simulink model "huamo"  (R2014a)
settings: Solver=ode3  SolverMode=SingleTasking  StartTime=0.0  StopTime=10.0  RelTol=1e-3
PreLoadFcn:
  | waijung.modelPreload; % Required for working with Waijung Blockset. Do not remove.
undefined symbols (not defined in the file): ARM, dfilt, DiscIntNeverNeededParam, fdesignblkfcn, gcbh, Link, LQFP64, MDK, ST, STM32F405RG
libraries: simulink x33, stm32f4_io_lib x3, stm32f4_device_config_lib x2, dsparch4 x2
(part 6 of 6)

== system huamo/ from shangweiji/Enabled Subsystem1/If Action Subsystem1 ==
  Action Port : ActionPort  ActionType=else
  UART Tx : S-Function  Priority=1  FunctionName=stm32f4_usart  Parameters=configuration,uartmodule,transfer,baudrate,inputtype,outputtype,confstr,binheaderarray,binterminatorarray,asciiheader,asciiterminator,bindatalength,packetmode,varname,sampletime,sampletimestr,blockid  EnableBusSupport=off  mask(stm32f4_usart){configuration=Tx, uartmodule=1, baudrate=115200, databits=8, parity=No, stopbit=1, remaptxpin=Not used, remaprxpin=Not used, flowcontrol=None, remapctspin=Not used, remaprtspin=Not used, advanceoptions=off, rxbuffersize=512, txbuffersize=512, transfer=Non-Blocking, packetmode=Ascii, binheader='7E 7E', binterminator='03 03', porttype_double=0, porttype_single=0, porttype_int8=0, porttype_uint8=0, porttype_int16=0, porttype_uint16=0, porttype_int32=0, porttype_uint32=3, asciiformat='>>LED1 ON', rx_asciiterminator=CRLF (0x0D 0x0A - "\r\n"), tx_asciiterminator=CRLF (0x0D 0x0A - "\r\n"), storagename=<empty>, varname=, inputtype=[0 ], outputtype=[0], binheaderarray=[0], binterminatorarray=[0], bindatalength=0, asciiheader='>>LED1 ON\r\n', asciiterminator=[2 13 10], sampletime=1, sampletimestr=1, blockid=fromshangweijiEnabledSubsystem1IfActionSubsystem1UARTTx, confstr=[ "dummy", "0", "*", "*", "0", "*", "*", "0", "*", "*", "0", "*", "*", "2", "4", "7", "2", "4", "2", "512", "512", "2", "1", "115200", "8", "No", "1", "None", "USART1"], lastmodule=1}
      mask prompts: uartmodule "UART Module"; baudrate "Baud rate (bps)"; databits "Data bits"; stopbit "Stop bit"; remaptxpin "Tx Pin"; remaprxpin "Rx Pin"; flowcontrol "Hardware flow control"; remapctspin "HW Flow control, CTS Pin"; remaprtspin "HW Flow control, RTS Pin"; advanceoptions "Advance options"; rxbuffersize "Rx buffer size (bytes)"; txbuffersize "Tx buffer size (bytes)"; packetmode "Packet mode"; binheader "Binary header (example: '7E 7E')"; binterminator "Binary terminator (example: '03 03')"; porttype_double "Number of data port, type DOUBLE"; porttype_single "Number of data port, type SINGLE"; porttype_int8 "Number of data port, type INT8"; porttype_uint8 "Number of data port, type UINT8"; porttype_int16 "Number of data port, type INT16"; porttype_uint16 "Number of data port, type UINT16"; porttype_int32 "Number of data port, type INT32"; porttype_uint32 "Number of data port, type UINT32"; asciiformat "Ascii format"; rx_asciiterminator "End of packet"; tx_asciiterminator "End of packet"; storagename "Buffer"; varname "Var name"; inputtype "Input data type"; outputtype "Output data type"; binheaderarray "Binary header"; binterminatorarray "Binary terminator"; bindatalength "Binary data length"; asciiheader "Ascii header (printf format)"; asciiterminator "Ascii terminator"; sampletime "Sample time (sec)"; sampletimestr "Compiled sample time (sec) in string"; confstr "Configuration string"; lastmodule "Last module selected"
      mask help:
      | Data type for Ascii format
      | %u, %i, %d, %o, %x: uint32
      | %e, %g, %f: single
      | %c: int8
      mask init:
      | stm32f4_usart_callback('init');
      mask Help: web(fullfile(waijungdocroot,'stm32f4_usart_tx.htm'), '-browser')
      mask TypeOptions configuration: Setup | Tx | Rx
      mask Callback configuration: stm32f4_usart_callback('configuration');
      mask TypeOptions uartmodule: 1 | 2 | 3 | 4 | 5 | 6
      mask Callback uartmodule: stm32f4_usart_callback('uartmodule');
      mask Callback baudrate: stm32f4_usart_callback('baudrate');
      mask TypeOptions databits: 8
      mask TypeOptions parity: No | Odd | Even
      mask TypeOptions stopbit: 0.5 | 1 | 1.5 | 2
      mask TypeOptions remaptxpin: Not used | A9 | B6
      mask TypeOptions remaprxpin: Not used | A10 | B7
      mask TypeOptions flowcontrol: None | RTS | CTS | RTS/CTS
      mask Callback flowcontrol: stm32f4_usart_callback('flowcontrol');
      mask TypeOptions remapctspin: Not used | A11
      mask TypeOptions remaprtspin: Not used | A12
      mask Callback advanceoptions: stm32f4_usart_callback('advanceoptions');
      mask TypeOptions rxbuffersize: 16 | 32 | 64 | 128 | 256 | 512 | 1024 | 2048
      mask TypeOptions txbuffersize: 16 | 32 | 64 | 128 | 256 | 512 | 1024 | 2048
      mask TypeOptions transfer: Blocking | Non-Blocking
      mask Callback transfer: stm32f4_usart_callback('transfer');
      mask TypeOptions packetmode: Ascii | Binary | Binary Vector | String Buffer
      mask Callback packetmode: stm32f4_usart_callback('packetmode');
      mask Callback binheader: stm32f4_usart_callback('binheader');
      mask Callback binterminator: stm32f4_usart_callback('binterminator');
      mask Callback porttype_double: stm32f4_usart_callback('porttype');
      mask Callback porttype_single: stm32f4_usart_callback('porttype');
      mask Callback porttype_int8: stm32f4_usart_callback('porttype');
      mask Callback porttype_uint8: stm32f4_usart_callback('porttype');
      mask Callback porttype_int16: stm32f4_usart_callback('porttype');
      mask Callback porttype_uint16: stm32f4_usart_callback('porttype');
      mask Callback porttype_int32: stm32f4_usart_callback('porttype');
      mask Callback porttype_uint32: stm32f4_usart_callback('porttype');
      mask Callback asciiformat: stm32f4_usart_callback('asciiformat');
      mask TypeOptions rx_asciiterminator: CR (0x0D - "\r") | LF (0x0A - "\n") | CRLF (0x0D 0x0A - "\r\n")
      mask Callback rx_asciiterminator: stm32f4_usart_callback('rx_asciiterminator');
      mask TypeOptions tx_asciiterminator: CR (0x0D - "\r") | LF (0x0A - "\n") | CRLF (0x0D 0x0A - "\r\n") | None
      mask Callback tx_asciiterminator: stm32f4_usart_callback('tx_asciiterminator');
      mask TypeOptions storagename: <empty>
      mask Callback storagename: stm32f4_usart_callback('storagename');
      mask Callback varname: stm32f4_usart_callback('varname');
      mask Callback sampletime: stm32f4_usart_callback('sampletime');
      mask Callback sampletimestr: stm32f4_usart_callback('sampletimestr');
      mask Callback blockid: stm32f4_usart_callback('blockid');
      mask Display: text(0.5, 0.5, 'Module: USART1_Tx\nPacket: Ascii\nTransfer: Non-Blocking\nTs (sec): 1','ver','middle','hor','center');

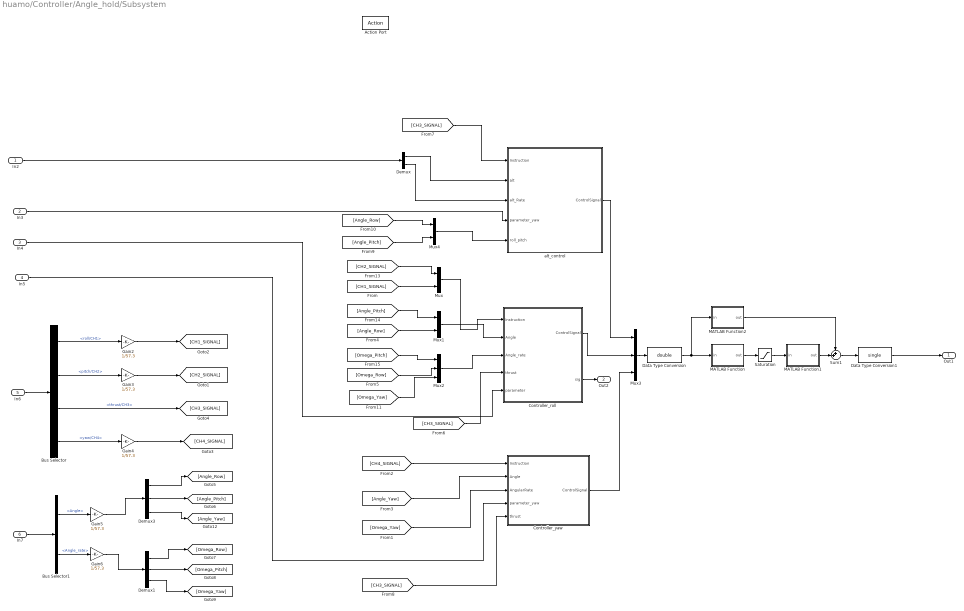
== system huamo/Controller/Angle_hold/Subsystem ==
  In2 : Inport
  In3 : Inport  Port=2
  In4 : Inport  Port=3
  In5 : Inport  Port=4
  In6 : Inport  Port=5
  In7 : Inport  Port=6
  Action Port : ActionPort  ActionType=then
  Bus Selector : BusSelector  OutputSignals=roll/CH1,pitch/CH2,thrust/CH3,yaw/CH4
  Bus Selector1 : BusSelector  OutputSignals=Angle,Angle_rate
  Controller_roll : Subsystem
  Controller_yaw : Subsystem
  Data Type Conversion : DataTypeConversion  OutDataTypeStr=double
  Data Type Conversion1 : DataTypeConversion  OutDataTypeStr=single
  Demux : Demux  Outputs=2
  Demux1 : Demux  Outputs=3
  Demux3 : Demux  Outputs=3
  Gain{2..6} (5 alike) : Gain  Gain=1/57.3
  MATLAB Function : MATLAB Function  TreatAsAtomicUnit=on
  MATLAB Function1 : MATLAB Function  TreatAsAtomicUnit=on
  MATLAB Function2 : MATLAB Function  TreatAsAtomicUnit=on
  Mux : Mux  Inputs=2
  Mux1 : Mux  Inputs=2
  Mux2 : Mux  Inputs=3
  Mux3 : Mux  Inputs=3
  Mux4 : Mux  Inputs=2
  Saturation : Saturate  UpperLimit=5.1564e+05  LowerLimit=8.0569e+03
  Sum1 : Sum  Inputs=++|
  alt_control : Subsystem
  Out1 : Outport
  Out2 : Outport  Port=2
  wires:
  In7/1 -> Bus Selector1/1
  Bus Selector1/2 -> Gain6/1  "<Angle_rate>"
  Bus Selector/4 -> Gain4/1  "<yaw/CH4>"
  In6/1 -> Bus Selector/1
  Bus Selector/2 -> Gain3/1  "<pitch/CH2>"
  Bus Selector/1 -> Gain2/1  "<roll/CH1>"
  Bus Selector/3 -> [CH3_SIGNAL]  "<thrust/CH3>"
  Demux3/1 -> [Angle_Row]
  Demux3/2 -> [Angle_Pitch]
  Demux1/1 -> [Omega_Row]
  Demux1/2 -> [Omega_Pitch]
  Demux1/3 -> [Omega_Yaw]
  Bus Selector1/1 -> Gain5/1  "<Angle>"
  Mux/1 -> Controller_roll/1(Instruction)
  Mux2/1 -> Controller_roll/3(Angle_rate)
  Mux1/1 -> Controller_roll/2(Angle)
  Demux3/3 -> [Angle_Yaw]
  [CH4_SIGNAL] -> Controller_yaw/1(Instruction)
  Gain2/1 -> [CH1_SIGNAL]
  Gain3/1 -> [CH2_SIGNAL]
  Gain4/1 -> [CH4_SIGNAL]
  Gain5/1 -> Demux3/1
  Gain6/1 -> Demux1/1
  Controller_yaw/1(ControlSignal) -> Mux3/3
  [Omega_Yaw] -> Controller_yaw/3(AngularRate)
  [Angle_Yaw] -> Controller_yaw/2(Angle)
  Mux3/1 -> Data Type Conversion/1
  MATLAB Function/1(out) -> Saturation/1
  Data Type Conversion/1 -> MATLAB Function2/1(in), MATLAB Function/1(in)
  Data Type Conversion1/1 -> Out1/1
  Saturation/1 -> MATLAB Function1/1(in)
  In4/1 -> Controller_roll/5(parameter)
  In5/1 -> Controller_yaw/4(parameter_yaw)
  [CH3_SIGNAL] -> Controller_roll/4(thrust)
  [CH3_SIGNAL] -> Controller_yaw/5(thrust)
  In2/1 -> Demux/1
  Demux/1 -> alt_control/2(alt)
  Demux/2 -> alt_control/3(alt_Rate)
  In3/1 -> alt_control/4(parameter_yaw)
  [Angle_Row] -> Mux4/1
  [Angle_Pitch] -> Mux4/2
  Mux4/1 -> alt_control/5(roll_pitch)
  alt_control/1(ControlSignal) -> Mux3/1
  [Omega_Row] -> Mux2/2
  [Omega_Pitch] -> Mux2/1
  [Angle_Row] -> Mux1/2
  [Angle_Pitch] -> Mux1/1
  [CH1_SIGNAL] -> Mux/2
  [CH2_SIGNAL] -> Mux/1
  Controller_roll/1(ControlSignal) -> Mux3/2
  Sum1/1 -> Data Type Conversion1/1
  MATLAB Function1/1(out) -> Sum1/2
  MATLAB Function2/1(out) -> Sum1/1
  Controller_roll/2(sig) -> Out2/1
  [CH3_SIGNAL] -> alt_control/1(Instruction)
  [Omega_Yaw] -> Mux2/3

== system huamo/Controller/Velocity_Damper1/Altitude_calculation ==
  Accelerometer : Inport
  Barometer : Inport  Port=2
  Basic_altitude : Inport  Port=3
  Enable : EnablePort
  Data Type Conversion : DataTypeConversion  OutDataTypeStr=single
  Data Type Conversion1 : DataTypeConversion  OutDataTypeStr=single
  Demux : Demux  Outputs=3
  Digital Clock : DigitalClock  SampleTime=-1
  Discrete-Time Integrator : DiscreteIntegrator  gainval=1  SampleTime=-1  ICPrevOutput=DiscIntNeverNeededParam  ICPrevScaledInput=DiscIntNeverNeededParam
  Discrete-Time Integrator1 : DiscreteIntegrator  SampleTime=-1  ICPrevOutput=DiscIntNeverNeededParam  ICPrevScaledInput=DiscIntNeverNeededParam
  Divide : Product  Inputs=**
  Gain2 : Gain  Gain=0.45
  Gain3 : Gain  Gain=0.65
  MATLAB Function : MATLAB Function  TreatAsAtomicUnit=on
  Rate Transition : RateTransition
  Sum{1..4} (4 alike) : Sum  Inputs=|+-
  Terminator : Terminator
  Terminator1 : Terminator
  Out1 : Outport
  wires:
  Rate Transition/1 -> Sum1/2
  Discrete-Time Integrator1/1 -> Out1/1, Sum1/1
  Discrete-Time Integrator/1 -> Sum3/1
  Sum4/1 -> Discrete-Time Integrator/1
  Sum3/1 -> Discrete-Time Integrator1/1
  Sum2/1 -> Rate Transition/1
  Demux/3 -> Sum4/1
  Barometer/1 -> Sum2/1
  Basic_altitude/1 -> Data Type Conversion/1
  Data Type Conversion/1 -> Sum2/2
  Accelerometer/1 -> Demux/1
  Demux/1 -> Terminator/1
  Demux/2 -> Terminator1/1
  Gain2/1 -> Sum4/2
  Gain3/1 -> Sum3/2
  Divide/1 -> Gain2/1, Gain3/1
  Sum1/1 -> Divide/1
  MATLAB Function/1(y) -> Data Type Conversion1/1
  Digital Clock/1 -> MATLAB Function/1(u)
  Data Type Conversion1/1 -> Divide/2

== system huamo/Controller/Velocity_Damper1/Controller ==
  In1 : Inport
  Discrete Derivative : simulink/Discrete/Discrete Derivative  gainval=1.0  ICPrevScaledInput=0.0  InputProcessing=Inherited  OutMin=[]  OutMax=[]  OutDataType=fixdt(1, 16)  OutScaling=2^-10  DoSatur=off
  Discrete FIR Filter : DiscreteFir  SampleTime=0.05
  Saturation : Saturate  UpperLimit=2  LowerLimit=-2
  Out1 : Outport
  wires:
  In1/1 -> Discrete Derivative/1
  Discrete Derivative/1 -> Discrete FIR Filter/1
  Saturation/1 -> Out1/1
  Discrete FIR Filter/1 -> Saturation/1

== system huamo/Controller/Velocity_Damper1/Horizontal_velocity ==
  note: To get true velocity ,the output of the loop needs to multiply -1
  In1 : Inport
  Dead Zone : DeadZone  LowerValue=-0.15  UpperValue=0.15  SaturateOnIntegerOverflow=on
  Demux : Demux  Outputs=3
  Discrete-Time Integrator : DiscreteIntegrator  SampleTime=-1  ICPrevOutput=DiscIntNeverNeededParam  ICPrevScaledInput=DiscIntNeverNeededParam
  Gain : Gain  Gain=0.5
  Gain2 : Gain  Gain=20
  Gain4 : Gain  Gain=-1
  Saturation : Saturate  UpperLimit=20  LowerLimit=-20
  Sum : Sum  Inputs=|+-
  Terminator : Terminator
  Out1 : Outport
  Out2 : Outport  Port=2
  wires:
  Demux/3 -> Terminator/1
  Demux/1 -> Out1/1
  Sum/1 -> Discrete-Time Integrator/1
  Gain/1 -> Sum/2
  Demux/2 -> Out2/1
  Discrete-Time Integrator/1 -> Gain4/1, Gain/1
  In1/1 -> Sum/1
  Dead Zone/1 -> Gain2/1
  Gain2/1 -> Saturation/1
  Saturation/1 -> Demux/1
  Gain4/1 -> Dead Zone/1

== system huamo/Controller/Velocity_Damper1/If Action Subsystem ==
  Action Port : ActionPort  ActionType=then
  Constant : Constant
  Out1 : Outport  InitialOutput=0
  wires:
  Constant/1 -> Out1/1

== system huamo/Controller/Velocity_Damper1/accb_to_acce ==
  angle : Inport
  accel : Inport  Port=2
  bias_acc : Inport  Port=3
  body axis to earth axis : MATLAB Function  TreatAsAtomicUnit=on
  Out1 : Outport
  wires:
  angle/1 -> body axis to earth axis/1(angle)
  accel/1 -> body axis to earth axis/2(acc_body)
  bias_acc/1 -> body axis to earth axis/3(bia_acc)
  body axis to earth axis/1(acc_earth) -> Out1/1

== system huamo/Controller/Velocity_Damper2/Controller ==
  In1 : Inport
  Discrete Derivative : simulink/Discrete/Discrete Derivative  gainval=1.0  ICPrevScaledInput=0.0  InputProcessing=Inherited  OutMin=[]  OutMax=[]  OutDataType=fixdt(1, 16)  OutScaling=2^-10  DoSatur=off
  Lowpass Filter : Subsystem  DialogController=fdesignblkfcn  InitFcn=fdesignblkfcn(gcbh, {'InitFcn'});  mask(Lowpass Filter){}
      mask help: Design a lowpass filter
      settings: CopyFcn=fdesignblkfcn(gcbh, {'CopyFcn'});
      mask Help: helpview(mapfilelocation('dsp'), 'dsplowpassfilter');
      mask Display: disp('Lowpass')
  Saturation : Saturate  UpperLimit=2  LowerLimit=-2
  Out1 : Outport
  wires:
  In1/1 -> Discrete Derivative/1
  Discrete Derivative/1 -> Lowpass Filter/1(In)
  Saturation/1 -> Out1/1
  Lowpass Filter/1(Out) -> Saturation/1

== system huamo/Controller/Velocity_Damper2/Lowpass Filter ==
  In : Inport
  Generated Filter Block : dsparch4/Biquad Filter  Tag=BlockMethodSubSystem  IIRFiltStruct=Direct form II  CoeffSource=Specify via dialog  BiQuadCoeffs=[0.31598662750883372 0.36803820725630498 0.31598662750883377 1 -1.8265775363780477 0.840471451002894]  a0Flag=Warning  IC=0  ICnum=0  ICden=0  InputProcessing=Columns as channels (frame based)  denAccumFracLength=30  denProdOutputFracLength=30  secondMemoryFracLength=15  roundingMode=Floor  overflowMode=off  ScaleValues=[0.013893755370815749;1]  optimizeScaleValues=off  ScaleValueMode=Specify via input port (g)  scaleValueFracLength=14  FilterSource=Specify via dialog  dfiltObjectName=dfilt.df2tsos([1 0.3 0.4],[1 0.1 0.2])
  Out : Outport
  wires:
  In/1 -> Generated Filter Block/1
  Generated Filter Block/1 -> Out/1

== system huamo/IMU/Cal/bu ma ==
  In1 : Inport
  Bitwise Operator : simulink/Logic and Bit Operations/Bitwise Operator  logicop=NOT  UseBitMask=off  BitMask=bin2dec('11011001')  BitMaskRealWorld=Stored Integer
  Bitwise Operator1 : simulink/Logic and Bit Operations/Bitwise Operator  logicop=OR  UseBitMask=on  BitMask=bin2dec('1000000000000000')  BitMaskRealWorld=Stored Integer
  Bitwise Operator2 : simulink/Logic and Bit Operations/Bitwise Operator  logicop=AND  UseBitMask=on  BitMask=bin2dec('1000000000000000')  BitMaskRealWorld=Stored Integer
  Constant : Constant  OutDataTypeStr=int16
  Sum : Sum  Inputs=|++
  Switch : Switch  Criteria=u2 > Threshold
  Out1 : Outport
  wires:
  Switch/1 -> Out1/1
  Bitwise Operator/1 -> Bitwise Operator1/1
  Constant/1 -> Sum/2
  Bitwise Operator1/1 -> Sum/1
  Sum/1 -> Switch/1
  In1/1 -> Bitwise Operator/1, Switch/3, Bitwise Operator2/1
  Bitwise Operator2/1 -> Switch/2

== system huamo/IMU/Cal/bu ma1 ==
  In1 : Inport
  Bitwise Operator : simulink/Logic and Bit Operations/Bitwise Operator  logicop=NOT  UseBitMask=off  BitMask=bin2dec('11011001')  BitMaskRealWorld=Stored Integer
  Bitwise Operator1 : simulink/Logic and Bit Operations/Bitwise Operator  logicop=OR  UseBitMask=on  BitMask=bin2dec('1000000000000000')  BitMaskRealWorld=Stored Integer
  Bitwise Operator2 : simulink/Logic and Bit Operations/Bitwise Operator  logicop=AND  UseBitMask=on  BitMask=bin2dec('1000000000000000')  BitMaskRealWorld=Stored Integer
  Constant : Constant  OutDataTypeStr=int16
  Sum : Sum  Inputs=|++
  Switch : Switch  Criteria=u2 > Threshold
  Out1 : Outport
  wires:
  Switch/1 -> Out1/1
  Bitwise Operator/1 -> Bitwise Operator1/1
  Constant/1 -> Sum/2
  Bitwise Operator1/1 -> Sum/1
  Sum/1 -> Switch/1
  In1/1 -> Bitwise Operator/1, Switch/3, Bitwise Operator2/1
  Bitwise Operator2/1 -> Switch/2

== system huamo/IMU/Cal/bu ma2 ==
  In1 : Inport
  Bitwise Operator : simulink/Logic and Bit Operations/Bitwise Operator  logicop=NOT  UseBitMask=off  BitMask=bin2dec('11011001')  BitMaskRealWorld=Stored Integer
  Bitwise Operator1 : simulink/Logic and Bit Operations/Bitwise Operator  logicop=OR  UseBitMask=on  BitMask=bin2dec('1000000000000000')  BitMaskRealWorld=Stored Integer
  Bitwise Operator2 : simulink/Logic and Bit Operations/Bitwise Operator  logicop=AND  UseBitMask=on  BitMask=bin2dec('1000000000000000')  BitMaskRealWorld=Stored Integer
  Constant : Constant  OutDataTypeStr=int16
  Sum : Sum  Inputs=|++
  Switch : Switch  Criteria=u2 > Threshold
  Out1 : Outport
  wires:
  Switch/1 -> Out1/1
  Bitwise Operator/1 -> Bitwise Operator1/1
  Constant/1 -> Sum/2
  Bitwise Operator1/1 -> Sum/1
  Sum/1 -> Switch/1
  In1/1 -> Bitwise Operator/1, Switch/3, Bitwise Operator2/1
  Bitwise Operator2/1 -> Switch/2

== system huamo/IMU/Cal/bu ma3 ==
  In1 : Inport
  Bitwise Operator : simulink/Logic and Bit Operations/Bitwise Operator  logicop=NOT  UseBitMask=off  BitMask=bin2dec('11011001')  BitMaskRealWorld=Stored Integer
  Bitwise Operator1 : simulink/Logic and Bit Operations/Bitwise Operator  logicop=OR  UseBitMask=on  BitMask=bin2dec('1000000000000000')  BitMaskRealWorld=Stored Integer
  Bitwise Operator2 : simulink/Logic and Bit Operations/Bitwise Operator  logicop=AND  UseBitMask=on  BitMask=bin2dec('1000000000000000')  BitMaskRealWorld=Stored Integer
  Constant : Constant  OutDataTypeStr=int16
  Sum : Sum  Inputs=|++
  Switch : Switch  Criteria=u2 > Threshold
  Out1 : Outport
  wires:
  Switch/1 -> Out1/1
  Bitwise Operator/1 -> Bitwise Operator1/1
  Constant/1 -> Sum/2
  Bitwise Operator1/1 -> Sum/1
  Sum/1 -> Switch/1
  In1/1 -> Bitwise Operator/1, Switch/3, Bitwise Operator2/1
  Bitwise Operator2/1 -> Switch/2

== system huamo/IMU/Cal/bu ma4 ==
  In1 : Inport
  Bitwise Operator : simulink/Logic and Bit Operations/Bitwise Operator  logicop=NOT  UseBitMask=off  BitMask=bin2dec('11011001')  BitMaskRealWorld=Stored Integer
  Bitwise Operator1 : simulink/Logic and Bit Operations/Bitwise Operator  logicop=OR  UseBitMask=on  BitMask=bin2dec('1000000000000000')  BitMaskRealWorld=Stored Integer
  Bitwise Operator2 : simulink/Logic and Bit Operations/Bitwise Operator  logicop=AND  UseBitMask=on  BitMask=bin2dec('1000000000000000')  BitMaskRealWorld=Stored Integer
  Constant : Constant  OutDataTypeStr=int16
  Sum : Sum  Inputs=|++
  Switch : Switch  Criteria=u2 > Threshold
  Out1 : Outport
  wires:
  Switch/1 -> Out1/1
  Bitwise Operator/1 -> Bitwise Operator1/1
  Constant/1 -> Sum/2
  Bitwise Operator1/1 -> Sum/1
  Sum/1 -> Switch/1
  In1/1 -> Bitwise Operator/1, Switch/3, Bitwise Operator2/1
  Bitwise Operator2/1 -> Switch/2

== system huamo/IMU/Cal/bu ma5 ==
  In1 : Inport
  Bitwise Operator : simulink/Logic and Bit Operations/Bitwise Operator  logicop=NOT  UseBitMask=off  BitMask=bin2dec('11011001')  BitMaskRealWorld=Stored Integer
  Bitwise Operator1 : simulink/Logic and Bit Operations/Bitwise Operator  logicop=OR  UseBitMask=on  BitMask=bin2dec('1000000000000000')  BitMaskRealWorld=Stored Integer
  Bitwise Operator2 : simulink/Logic and Bit Operations/Bitwise Operator  logicop=AND  UseBitMask=on  BitMask=bin2dec('1000000000000000')  BitMaskRealWorld=Stored Integer
  Constant : Constant  OutDataTypeStr=int16
  Sum : Sum  Inputs=|++
  Switch : Switch  Criteria=u2 > Threshold
  Out1 : Outport
  wires:
  Switch/1 -> Out1/1
  Bitwise Operator/1 -> Bitwise Operator1/1
  Constant/1 -> Sum/2
  Bitwise Operator1/1 -> Sum/1
  Sum/1 -> Switch/1
  In1/1 -> Bitwise Operator/1, Switch/3, Bitwise Operator2/1
  Bitwise Operator2/1 -> Switch/2

== system huamo/IMU/Cal/bu ma6 ==
  In1 : Inport
  Bitwise Operator : simulink/Logic and Bit Operations/Bitwise Operator  logicop=NOT  UseBitMask=off  BitMask=bin2dec('11011001')  BitMaskRealWorld=Stored Integer
  Bitwise Operator1 : simulink/Logic and Bit Operations/Bitwise Operator  logicop=OR  UseBitMask=on  BitMask=bin2dec('1000000000000000')  BitMaskRealWorld=Stored Integer
  Bitwise Operator2 : simulink/Logic and Bit Operations/Bitwise Operator  logicop=AND  UseBitMask=on  BitMask=bin2dec('1000000000000000')  BitMaskRealWorld=Stored Integer
  Constant : Constant  OutDataTypeStr=int16
  Sum : Sum  Inputs=|++
  Switch : Switch  Criteria=u2 > Threshold
  Out1 : Outport
  wires:
  Switch/1 -> Out1/1
  Bitwise Operator/1 -> Bitwise Operator1/1
  Constant/1 -> Sum/2
  Bitwise Operator1/1 -> Sum/1
  Sum/1 -> Switch/1
  In1/1 -> Bitwise Operator/1, Switch/3, Bitwise Operator2/1
  Bitwise Operator2/1 -> Switch/2

== system huamo/Controller/Angle_hold/Subsystem/Controller_roll ==
  Instruction : Inport
  Angle : Inport  Port=2
  Angle_rate : Inport  Port=3
  thrust : Inport  Port=4
  parameter : Inport  Port=5
  Data Type Conversion : DataTypeConversion  OutDataTypeStr=single
  Data Type Conversion8 : DataTypeConversion  OutDataTypeStr=double
  Mux1 : Mux  Inputs=5
  Saturation : Saturate  UpperLimit=0.8  LowerLimit=-0.8
  attitude_control : MATLAB Function  TreatAsAtomicUnit=on
  ControlSignal : Outport
  sig : Outport  Port=2
  wires:
  Data Type Conversion/1 -> Saturation/1
  Saturation/1 -> ControlSignal/1
  attitude_control/1(out) -> sig/1, Data Type Conversion/1
  Data Type Conversion8/1 -> attitude_control/1(in)
  Instruction/1 -> Mux1/1
  Angle/1 -> Mux1/2
  Angle_rate/1 -> Mux1/3
  thrust/1 -> Mux1/4
  parameter/1 -> Mux1/5
  Mux1/1 -> Data Type Conversion8/1

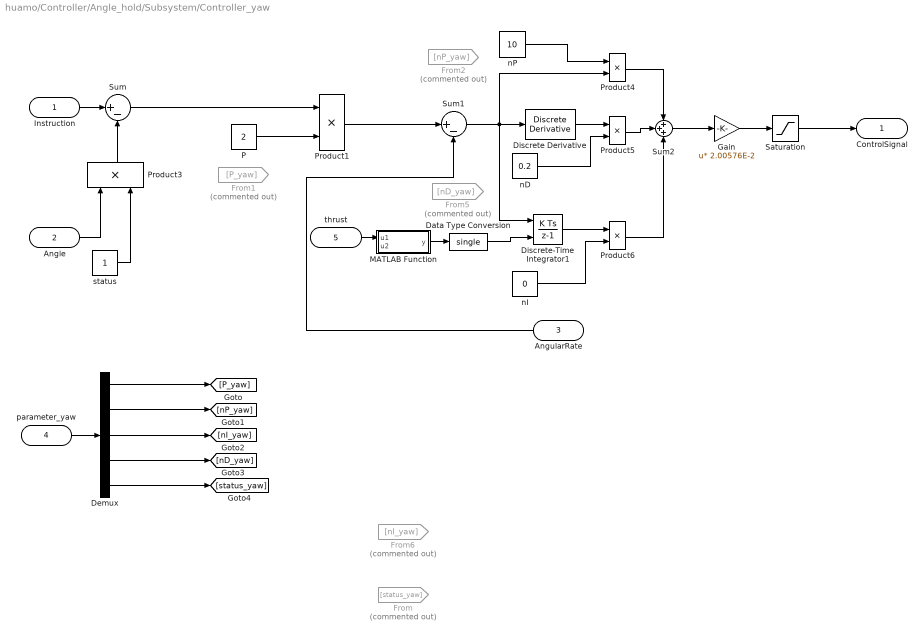
== system huamo/Controller/Angle_hold/Subsystem/Controller_yaw ==
  Instruction : Inport
  Angle : Inport  Port=2
  AngularRate : Inport  Port=3
  parameter_yaw : Inport  Port=4
  thrust : Inport  Port=5
  Data Type Conversion : DataTypeConversion  OutDataTypeStr=single
  Demux : Demux  Outputs=5
  Discrete Derivative : simulink/Discrete/Discrete Derivative  gainval=1.0  ICPrevScaledInput=0.01  InputProcessing=Inherited  OutMin=[]  OutMax=[]  OutDataType=fixdt(1, 16)  OutScaling=2^-10  DoSatur=off
  Discrete-Time Integrator1 : DiscreteIntegrator  ExternalReset=level  SampleTime=-1  LimitOutput=on  UpperSaturationLimit=2  LowerSaturationLimit=-2  ICPrevOutput=DiscIntNeverNeededParam  ICPrevScaledInput=DiscIntNeverNeededParam
  From : From  Commented=on  GotoTag=status_yaw
  From1 : From  Commented=on  GotoTag=P_yaw
  From2 : From  Commented=on  GotoTag=nP_yaw
  From5 : From  Commented=on  GotoTag=nD_yaw
  From6 : From  Commented=on  GotoTag=nI_yaw
  Gain : Gain  Gain=2.00576E-2  Multiplication=Matrix(u*K)  OutDataTypeStr=single
  MATLAB Function : MATLAB Function  TreatAsAtomicUnit=on
  P : Constant  Value=2  OutDataTypeStr=single
  Product{1,3..6} (5 alike) : Product
  Saturation : Saturate  UpperLimit=0.2  LowerLimit=-0.2
  Sum : Sum  Inputs=|+-
  Sum1 : Sum  Inputs=|+-  OutDataTypeStr=double
  Sum2 : Sum  Inputs=+++
  nD : Constant  Value=0.2  OutDataTypeStr=single
  nI : Constant  Value=0  OutDataTypeStr=single
  nP : Constant  Value=10  OutDataTypeStr=single
  status : Constant  OutDataTypeStr=single
  ControlSignal : Outport
  wires:
  Instruction/1 -> Sum/1
  Sum/1 -> Product1/1
  Sum1/1 -> Discrete Derivative/1, Discrete-Time Integrator1/1, Product4/2
  Angle/1 -> Product3/1
  Product3/1 -> Sum/2
  Sum2/1 -> Gain/1
  Discrete Derivative/1 -> Product5/1
  Discrete-Time Integrator1/1 -> Product6/1
  Product5/1 -> Sum2/2
  Product4/1 -> Sum2/1
  Product6/1 -> Sum2/3
  Product1/1 -> Sum1/1
  AngularRate/1 -> Sum1/2
  Gain/1 -> Saturation/1
  Saturation/1 -> ControlSignal/1
  parameter_yaw/1 -> Demux/1
  Demux/1 -> [P_yaw]
  Demux/2 -> [nP_yaw]
  Demux/3 -> [nI_yaw]
  Demux/4 -> [nD_yaw]
  Demux/5 -> [status_yaw]
  thrust/1 -> MATLAB Function/1(u1)
  MATLAB Function/1(y) -> Data Type Conversion/1
  Data Type Conversion/1 -> Discrete-Time Integrator1/2
  status/1 -> Product3/2
  nI/1 -> Product6/2
  nP/1 -> Product4/1
  P/1 -> Product1/2
  nD/1 -> Product5/2

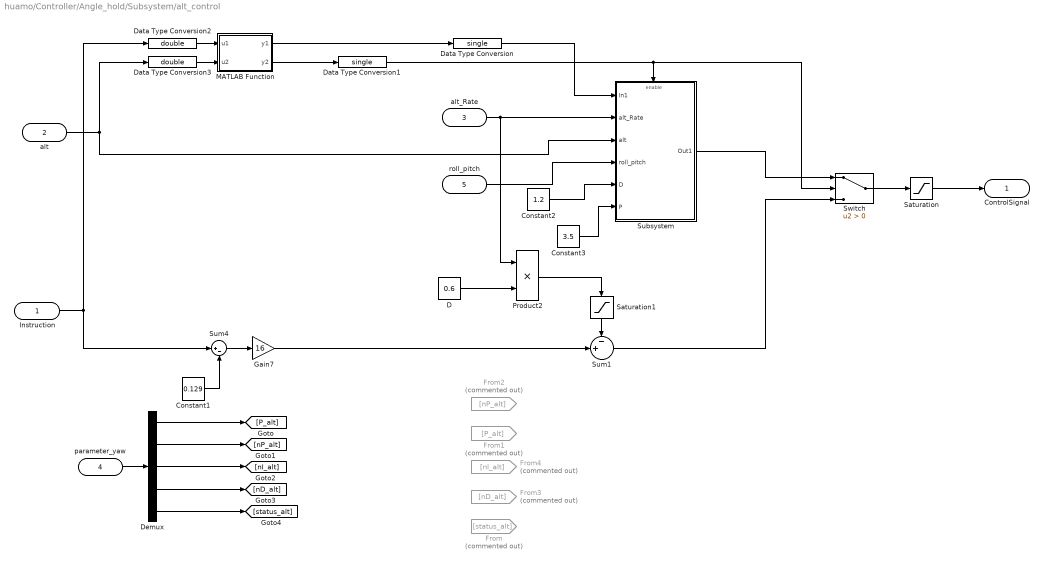
== system huamo/Controller/Angle_hold/Subsystem/alt_control ==
  Instruction : Inport
  alt : Inport  Port=2
  alt_Rate : Inport  Port=3
  parameter_yaw : Inport  Port=4
  roll_pitch : Inport  Port=5
  Constant1 : Constant  Value=0.129  OutDataTypeStr=single
  Constant2 : Constant  Value=1.2  OutDataTypeStr=single
  Constant3 : Constant  Value=3.5  OutDataTypeStr=single
  D : Constant  Value=0.6  OutDataTypeStr=single
  Data Type Conversion : DataTypeConversion  OutDataTypeStr=single
  Data Type Conversion1 : DataTypeConversion  OutDataTypeStr=single
  Data Type Conversion2 : DataTypeConversion  OutDataTypeStr=double
  Data Type Conversion3 : DataTypeConversion  OutDataTypeStr=double
  Demux : Demux  Outputs=5
  From : From  Commented=on  GotoTag=status_alt
  From1 : From  Commented=on  GotoTag=P_alt
  From2 : From  Commented=on  GotoTag=nP_alt
  From3 : From  Commented=on  GotoTag=nD_alt
  From4 : From  Commented=on  GotoTag=nI_alt
  Gain7 : Gain  Gain=16
  MATLAB Function : MATLAB Function  TreatAsAtomicUnit=on
  Product2 : Product
  Saturation : Saturate  UpperLimit=10  LowerLimit=0.272
  Saturation1 : Saturate  UpperLimit=1  LowerLimit=-1
  Subsystem : Subsystem
  Sum1 : Sum  Inputs=-+|  OutDataTypeStr=single
  Sum4 : Sum  Inputs=|+-
  Switch : Switch  Criteria=u2 > Threshold
  ControlSignal : Outport
  wires:
  Instruction/1 -> Sum4/1, Data Type Conversion2/1
  alt/1 -> Subsystem/3(alt), Data Type Conversion3/1
  Saturation/1 -> ControlSignal/1
  parameter_yaw/1 -> Demux/1
  Demux/1 -> [P_alt]
  Demux/2 -> [nP_alt]
  Demux/3 -> [nI_alt]
  Demux/4 -> [nD_alt]
  Demux/5 -> [status_alt]
  Constant1/1 -> Sum4/2
  Sum4/1 -> Gain7/1
  alt_Rate/1 -> Subsystem/2(alt_Rate), Product2/1
  roll_pitch/1 -> Subsystem/4(roll_pitch)
  MATLAB Function/1(y1) -> Data Type Conversion/1
  MATLAB Function/2(y2) -> Data Type Conversion1/1
  D/1 -> Product2/2
  Gain7/1 -> Sum1/2
  Product2/1 -> Saturation1/1
  Sum1/1 -> Switch/3
  Subsystem/1(Out1) -> Switch/1
  Switch/1 -> Saturation/1
  Data Type Conversion/1 -> Subsystem/1(In1)
  Data Type Conversion1/1 -> Subsystem/Enable, Switch/2
  Data Type Conversion2/1 -> MATLAB Function/1(u1)
  Data Type Conversion3/1 -> MATLAB Function/2(u2)
  Saturation1/1 -> Sum1/1
  Constant2/1 -> Subsystem/5(D)
  Constant3/1 -> Subsystem/6(P)

== system huamo/Controller/Velocity_Damper2/Controller/Lowpass Filter ==
  In : Inport
  Generated Filter Block : dsparch4/Biquad Filter  Tag=BlockMethodSubSystem  IIRFiltStruct=Direct form II  CoeffSource=Specify via dialog  BiQuadCoeffs=[0.31598662750883372 0.36803820725630498 0.31598662750883377 1 -1.8265775363780477 0.840471451002894]  a0Flag=Warning  IC=0  ICnum=0  ICden=0  InputProcessing=Columns as channels (frame based)  denAccumFracLength=30  denProdOutputFracLength=30  secondMemoryFracLength=15  roundingMode=Floor  overflowMode=off  ScaleValues=[0.013893755370815749;1]  optimizeScaleValues=off  ScaleValueMode=Specify via input port (g)  scaleValueFracLength=14  FilterSource=Specify via dialog  dfiltObjectName=dfilt.df2tsos([1 0.3 0.4],[1 0.1 0.2])
  Out : Outport
  wires:
  In/1 -> Generated Filter Block/1
  Generated Filter Block/1 -> Out/1

== system huamo/Controller/Angle_hold/Subsystem/alt_control/Subsystem ==
  In1 : Inport
  alt_Rate : Inport  Port=2
  alt : Inport  Port=3
  roll_pitch : Inport  Port=4
  D : Inport  Port=5
  P : Inport  Port=6
  Enable : EnablePort
  Constant : Constant  Value=10  OutDataTypeStr=single
  Constant1 : Constant  Value=0.43  OutDataTypeStr=single
  Data Type Conversion1 : DataTypeConversion  OutDataTypeStr=single
  Divide : Product  Inputs=*/  OutDataTypeStr=single
  Fcn : Fcn  Expr=cos(u(1))*cos(u(2))
  Product1 : Product
  Product2 : Product
  Product4 : Product
  Saturation1 : Saturate  UpperLimit=1.5  LowerLimit=-1.5
  Sum : Sum  Inputs=|+-
  Sum1 : Sum  Inputs=|+-  OutDataTypeStr=double
  Sum2 : Sum  Inputs=|++
  Out1 : Outport
  wires:
  alt_Rate/1 -> Product2/1
  Sum/1 -> Product1/1
  alt/1 -> Sum/2
  Product1/1 -> Sum1/1
  roll_pitch/1 -> Fcn/1
  Fcn/1 -> Data Type Conversion1/1
  Divide/1 -> Out1/1
  In1/1 -> Sum/1
  Data Type Conversion1/1 -> Divide/2
  Constant/1 -> Sum2/2
  Sum1/1 -> Sum2/1
  Constant1/1 -> Product4/2
  Sum2/1 -> Product4/1
  Product4/1 -> Divide/1
  Product2/1 -> Saturation1/1
  Saturation1/1 -> Sum1/2
  P/1 -> Product1/2
  D/1 -> Product2/2

== matlab function huamo/Receiver/Enabled Subsystem/MATLAB Function2 ==
  data: u input; y output
function y = fcn(u)
%#codegen
%输入范围为0.34~1.7，将其调整到1~2ms
    u=u/1.375+0.76;
    if (u>0.8)&&(u<2.1)
        y=u;
    else
        y=1.5;    
    end

== matlab function huamo/Receiver/Enabled Subsystem/MATLAB Function4 ==
  data: u input; y output
function y = fcn(u)
%#codegen
%输入范围为0.34~1.7，将其调整到1~2ms
    u=u/1.375+0.76;
    if (u>0.8)&&(u<2.1)
        y=u;
    else
        y=1.5;    
    end

== matlab function huamo/Controller/Angle_hold/Subsystem/MATLAB Function ==
  data: in input; out output
function out = fcn(in)
b= 8.7838E-6;       % [N.s2] thrust factor in hover
d= 7.5E-7;         % [Nm.s2] drag factor in hover
U=zeros(1,4);
U(1)=in(1);
U(2)=0;
U(3)=0;
U(4)=in(4);

mapmat=[ b  b b  b; 
         0 -b 0  b;
        -b  0 b  0;
         d -d d -d];    % thrust and drag coefficients matrix (for hover)
     
% Omd=sqrt(inv(mapmat)*U');   % desired prop speeds [rad/s]

% bin=(Omd+shi)/slo;  % setpoint to be sent to motor modules
bin=inv(mapmat)*U';
% Only for test
out=bin; % [dec]

== matlab function huamo/Receiver/Enabled Subsystem/MATLAB Function1 ==
  data: u input; y output
function y = fcn(u)
%#codegen
%输入范围为0.34~1.7，将其调整到1~2ms
    u=u/1.375+0.76;
    if (u>0.8)&&(u<2.1)
        y=u;
    else 
        y=1.5;    
    end

== matlab function huamo/Controller/Angle_hold/Subsystem/MATLAB Function1 ==
  data: in input; out output
function out = fcn(in)
bin=sqrt(in);
% Only for test
out=bin/(12*74.8);

== matlab function huamo/Controller/Angle_hold/Subsystem/Controller_yaw/MATLAB Function ==
  data: u1 input; y output; u2 input
function y = fcn(u1,u2)
%#codegen
    y=1;
    if u1>0.3            %if thrust>20%,enable integrator
        y=0;
    elseif u2<5         %if delta angle<5,enable integrator
        y=0;
    end

== matlab function huamo/Controller/Angle_hold/Subsystem/alt_control/MATLAB Function ==
  data: u1 input; y1 output; u2 input; y2 output
function [y1,y2] = fcn(u1,u2)
%#codegen
    persistent  a count;
    if isempty(a) 
        a=0;
    end
    if isempty(count)
        count=0;
    end
if (u1>0.35&&u1<0.45)&&count==0
    a=u2;
    count=1;
elseif u1<=0.35&&count==1
    count=0;
    a=0;
elseif u1>=0.45&&count==1
    count=0;
    a=0;
else
    count=0;
    a=0;
end
    y1=a;
    y2=count;

== matlab function huamo/Receiver/Enabled Subsystem/MATLAB Function3 ==
  data: u input; y output
function y = fcn(u)
%#codegen
%输入范围为0.34~1.7，将其调整到1~2ms
    u=u/1.375+0.75;
    if (u>1)&&(u<2.1)
        y=u;
    else
        y=1;
    end

== matlab function huamo/Controller/Angle_hold/Subsystem/MATLAB Function2 ==
  data: in input; out output
function out = fcn(in)
% b= 8.7838E-6;       % [N.s2] thrust factor in hover
% d= 7.5E-7;         % [Nm.s2] drag factor in hover
b=1;
d=1;
U=zeros(1,4);
U(1)=0;
U(2)=in(2);
U(3)=in(3);
U(4)=0;

mapmat=[ b  b b  b; 
         0 -b 0  b;
        -b  0 b  0;
         d -d d -d];    % thrust and drag coefficients matrix (for hover)
     
% Omd=sqrt(inv(mapmat)*U');   % desired prop speeds [rad/s]

% bin=(Omd+shi)/slo;  % setpoint to be sent to motor modules
bin=inv(mapmat)*U';
% Only for test
out=bin/2; % [dec]

== matlab function huamo/Controller/MATLAB Function ==
  data: u1 input; y output; u2 input
function y = fcn(u1,u2)
%#codegen
persistent status;
  if isempty(status)
      status=0;
  end
  if u1<0.1&&u2<-160
      status=1;
  elseif u1<0.1&&u2>160
      status=0;
  end
y = status;

== matlab function huamo/Controller/Angle_hold/Subsystem/Controller_roll/attitude_control ==
  data: in input; out output
% BECAUSE THE PROGRAM IS LICENSED FREE OF CHARGE, THERE IS NO WARRANTY
% FOR THE PROGRAM, TO THE EXTENT PERMITTED BY APPLICABLE LAW.  EXCEPT WHEN
% OTHERWISE STATED IN WRITING THE COPYRIGHT HOLDERS AND/OR OTHER PARTIES
% PROVIDE THE PROGRAM "AS IS" WITHOUT WARRANTY OF ANY KIND, EITHER EXPRESSED
% OR IMPLIED, INCLUDING, BUT NOT LIMITED TO, THE IMPLIED WARRANTIES OF
% MERCHANTABILITY AND FITNESS FOR A PARTICULAR PURPOSE.  THE ENTIRE RISK AS
% TO THE QUALITY AND PERFORMANCE OF THE PROGRAM IS WITH YOU.  SHOULD THE
% PROGRAM PROVE DEFECTIVE, YOU ASSUME THE COST OF ALL NECESSARY SERVICING,
% REPAIR OR CORRECTION.
% 
%   12. IN NO EVENT UNLESS REQUIRED BY APPLICABLE LAW OR AGREED TO IN WRITING
% WILL ANY COPYRIGHT HOLDER, OR ANY OTHER PARTY WHO MAY MODIFY AND/OR
% REDISTRIBUTE THE PROGRAM AS PERMITTED ABOVE, BE LIABLE TO YOU FOR DAMAGES,
% INCLUDING ANY GENERAL, SPECIAL, INCIDENTAL OR CONSEQUENTIAL DAMAGES ARISING
% OUT OF THE USE OR INABILITY TO USE THE PROGRAM (INCLUDING BUT NOT LIMITED
% TO LOSS OF DATA OR DATA BEING RENDERED INACCURATE OR LOSSES SUSTAINED BY
% YOU OR THIRD PARTIES OR A FAILURE OF THE PROGRAM TO OPERATE WITH ANY OTHER
% PROGRAMS), EVEN IF SUCH HOLDER OR OTHER PARTY HAS BEEN ADVISED OF THE
% POSSIBILITY OF SUCH DAMAGES.

% Rotations control function
% INPUT: state, (phi,theta,psi)(ref)
% OUTPUT: desired prop speeds

function out = fcn(in)
%#codegen
% global file for parameters
persistent count;
  if isempty(count)
      count=0;
  end
persistent x1_1;
  if isempty(x1_1)
      x1_1=0;
  end
persistent x2_1;
 if isempty(x2_1)
      x2_1=0;
 end
 U=zeros(2,1);
Ixx = 9.5012E-3;	%// [kg.m2]    
Iyy = 9.5012E-3;	%// [kg.m2]
Izz = 2.0057E-2;	%// [kg.m2]
%***** Rotor inertia *****/
sp= 0.01; % [s] sampling period only used to compute YiA term in dinamica.m
%***** Arm length *****/
L= 0.232; 			%// [m]

%***** Total mass *****/
m = 0.85;	%// [kg]

% ********* Operational Conditions *********
pitchd=in(1);   % desired PITCH angle [rad]
rolld=in(2);   % desired ROLL angle [rad]
pitch=in(3);
roll=in(4);     % [rad]
dotpitch=in(5);
dotroll=in(6);  % [rad/s]
dotyaw=in(7);
signal=in(8);
lamd=in(9);
kp=in(10);
kps=in(11);
s=in(12);
if signal>0.2

% ******************************************************** CONTROL ******************************************************** 

dotrolld = 0;     
dotpitchd = 0;

% ********* +滑模参数roll**************
lamdaroll=6.5;
kproll=17;
kpsroll=10;
deltaroll=0.05;
% ********* + 滑模参数pitch **************
lamdapitch=6.5;
kppitch=17;
kpspitch=10;
deltapitch=0.05;

intmax=5;
eroll=rolld-roll;
epitch=pitchd-pitch;
e1=2*kproll*eroll;  % roll error
e3=2*kppitch*epitch;  % pitch error

x1=x1_1+eroll*sp;  % integrator
x2=x2_1+epitch*sp;  % integrator
% if abs(eroll)>0.17
%     x1=0;
% end
% if abs(epitch)>0.17
%     x2=0;
% end
if x1>intmax
    x1=intmax;
elseif x1<-intmax
    x1=-intmax;
end
if x2>intmax
    x2=intmax;
elseif x2<-intmax
    x2=-intmax;
end

% ********* sliding surface **************
sroll=-1*dotroll+lamdaroll*eroll +kproll*x1;
spitch=-1*dotpitch+lamdapitch*epitch +kppitch*x2;
% ********* r2  **************
 if sroll<=-deltaroll
      r2=-deltaroll;
   elseif (sroll>=deltaroll)
      r2=deltaroll;
   else
      r2=sroll;
  end
% ********* r3  **************
if(spitch<=-1*deltapitch)
    r3=-1*deltapitch;
elseif (spitch>=deltapitch)
    r3=deltapitch;
else
    r3=spitch;
end

% Coconut controller

U(2)=(Ixx/L)*(e1-lamdaroll*dotroll-((Iyy-Izz)/Ixx)*dotpitch*dotyaw) + kpsroll*Ixx*r2;
U(1)=(Iyy/L)*(e3-lamdapitch*dotpitch-((Izz-Ixx)/Iyy)*dotroll*dotyaw) + kpspitch*Iyy*r3;
% update integrator
x1_1=x1;
x2_1=x2;
else
    x1_1=0;
    x2_1=0;
    U(1)=0;
    U(2)=0;
end
% Outputs
out=U;

== matlab function huamo/Controller/Velocity_Damper1/Altitude_calculation/MATLAB Function ==
  data: u input; y output
function y = fcn(u)
%#codegen
    if u<3
        y=1;
    else
        y=1;
    end

== matlab function huamo/Controller/Velocity_Damper1/Get_initial_altitude ==
  data: h input; y output; t input
function y = fcn(h,t)
%#codegen
    persistent a count;
    if isempty(a)
        a=0;
    end
    if isempty(count)
        count=0;
    end
    if (t<2)&&(t>0.75)
        a=a+double(h);
        count=count+1;
    end
    if t>=2
        y=a/count;
    else
        y=0;
    end

== matlab function huamo/Controller/Velocity_Damper1/MATLAB Function ==
  data: u1 input; y output; u2 input
function y = fcn(u1,u2)
%#codegen
persistent altitude_basic count;
  if isempty(altitude_basic)
      altitude_basic=0;
  end
  if isempty(count)
      count=0;
  end
if u1==1&&count==0
   count=1;
   altitude_basic=u2; 
elseif u1==0&&count==1
    count=0;
end
y = u2-altitude_basic;

== matlab function huamo/Controller/Velocity_Damper1/accb_to_acce/body axis to earth axis ==
  data: angle input; acc_earth output; acc_body input; bia_acc input
function acc_earth = fcn(angle, acc_body, bia_acc)
%#codegen
    angle_row  =angle(1);
    angle_pitch=angle(2);
    %angle_yaw  =angle(3);
    a1=acc_body(1);
    a2=acc_body(2);
    
    acc_body(1)=acc_body(1)*(-1);
    acc_body(2)=acc_body(2)*(-1);
    acc_body(3)=acc_body(3)*(-1);
    
    angle_yaw=0;
    
    A11=cosd(angle_pitch)*cosd(angle_yaw);
    A12=sind(angle_row)*sind(angle_pitch)*cosd(angle_yaw)-cosd(angle_row)*sind(angle_yaw);
    A13=cosd(angle_row)*sind(angle_pitch)*cosd(angle_yaw)+sind(angle_row)*sind(angle_yaw);
    
    A21=cosd(angle_pitch)*sind(angle_yaw);
    A22=sind(angle_row)*sind(angle_pitch)*sind(angle_yaw)+cosd(angle_row)*cosd(angle_yaw);
    A23=cosd(angle_row)*sind(angle_pitch)*sind(angle_yaw)-sind(angle_row)*cosd(angle_yaw);
    
    A31=-sind(angle_pitch);
    A32=sind(angle_row)*cosd(angle_pitch);
    A33=cosd(angle_row)*cosd(angle_pitch);
    
    T=[A11,A12,A13;A21,A22,A23;A31,A32,A33];
    
    a=T*acc_body;
    
    acc_earth=a';
    
    acc_earth(1)=acc_earth(1)-bia_acc(1);
    acc_earth(2)=acc_earth(2)-bia_acc(2);
    acc_earth(3)=acc_earth(3)-bia_acc(3);
acc_earth ;

== matlab function huamo/Controller/Velocity_Damper2/MATLAB Function ==
  data: u1 input; y output; u2 input
function y = fcn(u1,u2)
%#codegen
persistent altitude_basic count;
  if isempty(altitude_basic)
      altitude_basic=0;
  end
  if isempty(count)
      count=0;
  end
if u1==1&&count==0
   count=1;
   altitude_basic=u2; 
elseif u1==0&&count==1
    count=0;
end
y = u2-altitude_basic;
